simulink model "MS_QD2_QBP_joystick_R2023"  (R2023a)
settings: Solver=ode2  StartTime=0.0  StopTime=inf  FixedStep=0.001  RelTol=1e-3  EnableMultiTasking=on
undefined symbols (not defined in the file): Host, qc_get_step_size
libraries: quarc_library x67, simulink x9, simulink_extras x1
(part 2 of 2)

== system MS_QD2_QBP_joystick_R2023/MISSION SERVER LEADER FOLLOWER CONTROL/JOYSTICK_FRSKY/Pulse Check ==
  note: For this subsystem we will count the number of new pulses. The data can be considered enabled once the count of new signals has gone beyond 2. This will enable the Initializing and conditioning subsystem.
  new : Inport
  Compare : quarc_library/Logic Operations/Compare  operator=>=  output_data_type=boolean
      settings: SourceProductName=QUARC Targets
  Pulse Check : Constant
  "pulse count " : Subsystem  TreatAsAtomicUnit=on
  signal enable : Outport  InitialOutput=0  VectorParamsAs1DForOutWhenUnconnected=off
  wires:
  Compare/1 -> signal enable/1
  Pulse Check/1 -> Compare/2
  new/1 -> "pulse count "/Trigger
  "pulse count "/1(Number of Pulses) -> Compare/1

== system MS_QD2_QBP_joystick_R2023/MISSION SERVER LEADER FOLLOWER CONTROL/StopAllSignal/Subsystem ==
  Signal : Inport
  Delay : Delay  DelayLength=4
  Stop with Message : quarc_library/Sinks/Error Handling/Stop with Message  message_type=Fixed error message  message_icon=Error  message=QDrone Stopped, Stop all Models
  Threshold : quarc_library/Discontinuities/Threshold  operator=>=  param_src=Specify via dialog  threshold=0.5  duration=1
      settings: SourceProductName=QUARC Targets
  Threshold1 : quarc_library/Discontinuities/Threshold  operator=>=  param_src=Specify via dialog  threshold=0.5  duration=.3
      settings: SourceProductName=QUARC Targets
  Triggered Subsystem1 : Subsystem  TreatAsAtomicUnit=on
  Triggered Subsystem2 : Subsystem  TreatAsAtomicUnit=on
  Stop : Outport
  wires:
  Triggered Subsystem2/1(StopAllModels) -> Stop/1
  Signal/1 -> Threshold1/1, Threshold/1
  Threshold1/1 -> Triggered Subsystem2/Trigger
  Threshold/1 -> Triggered Subsystem1/Trigger, Delay/1
  Delay/1 -> Stop with Message/1

== system MS_QD2_QBP_joystick_R2023/MISSION SERVER LEADER FOLLOWER CONTROL/StopAllSignal/Subsystem1 ==
  Signal : Inport
  Delay : Delay  DelayLength=4
  Stop with Message : quarc_library/Sinks/Error Handling/Stop with Message  message_type=Fixed error message  message_icon=Error  message=Joystick triggers not back
  Threshold : quarc_library/Discontinuities/Threshold  operator=>=  param_src=Specify via dialog  threshold=0.5  duration=3
      settings: SourceProductName=QUARC Targets
  Threshold1 : quarc_library/Discontinuities/Threshold  operator=>=  param_src=Specify via dialog  threshold=0.5  duration=2
      settings: SourceProductName=QUARC Targets
  Triggered Subsystem1 : Subsystem  TreatAsAtomicUnit=on
  Triggered Subsystem2 : Subsystem  TreatAsAtomicUnit=on
  Stop : Outport
  wires:
  Triggered Subsystem2/1(StopAllModels) -> Stop/1
  Signal/1 -> Threshold1/1, Threshold/1
  Threshold1/1 -> Triggered Subsystem2/Trigger
  Threshold/1 -> Triggered Subsystem1/Trigger, Delay/1
  Delay/1 -> Stop with Message/1

== system MS_QD2_QBP_joystick_R2023/MISSION SERVER LEADER FOLLOWER CONTROL/StopAllSignal/Subsystem2 ==
  Signal : Inport
  Delay : Delay  DelayLength=4
  Stop with Message : quarc_library/Sinks/Error Handling/Stop with Message  message_type=Fixed error message  message_icon=Error  message=Not Tracking on start
  Threshold : quarc_library/Discontinuities/Threshold  operator=>=  param_src=Specify via dialog  threshold=0.5  duration=4
      settings: SourceProductName=QUARC Targets
  Threshold1 : quarc_library/Discontinuities/Threshold  operator=>=  param_src=Specify via dialog  threshold=0.5  duration=3
      settings: SourceProductName=QUARC Targets
  Triggered Subsystem1 : Subsystem  TreatAsAtomicUnit=on
  Triggered Subsystem2 : Subsystem  TreatAsAtomicUnit=on
  Stop : Outport
  wires:
  Triggered Subsystem2/1(StopAllModels) -> Stop/1
  Signal/1 -> Threshold1/1, Threshold/1
  Threshold1/1 -> Triggered Subsystem2/Trigger
  Threshold/1 -> Triggered Subsystem1/Trigger, Delay/1
  Delay/1 -> Stop with Message/1

== system MS_QD2_QBP_joystick_R2023/MISSION SERVER LEADER FOLLOWER CONTROL/StopAllSignal/Subsystem3 ==
  Signal : Inport
  Delay : Delay  DelayLength=4
  Stop with Message : quarc_library/Sinks/Error Handling/Stop with Message  message_type=Fixed error message  message_icon=Error  message=Emergency stop triggered
  Threshold : quarc_library/Discontinuities/Threshold  operator=>=  param_src=Specify via dialog  threshold=0.5  duration=2
      settings: SourceProductName=QUARC Targets
  Threshold1 : quarc_library/Discontinuities/Threshold  operator=>=  param_src=Specify via dialog  threshold=0.5  duration=.5
      settings: SourceProductName=QUARC Targets
  Triggered Subsystem1 : Subsystem  TreatAsAtomicUnit=on
  Triggered Subsystem2 : Subsystem  TreatAsAtomicUnit=on
  Stop : Outport
  wires:
  Triggered Subsystem2/1(StopAllModels) -> Stop/1
  Signal/1 -> Threshold1/1, Threshold/1
  Threshold1/1 -> Triggered Subsystem2/Trigger
  Threshold/1 -> Triggered Subsystem1/Trigger, Delay/1
  Delay/1 -> Stop with Message/1

== system MS_QD2_QBP_joystick_R2023/MISSION SERVER LEADER FOLLOWER CONTROL/StopAllSignal/Subsystem4 ==
  Signal : Inport
  Delay : Delay  DelayLength=4
  Stop with Message : quarc_library/Sinks/Error Handling/Stop with Message  message_type=Fixed error message  message_icon=Error  message=Autoland Triggered
  Threshold : quarc_library/Discontinuities/Threshold  operator=>=  param_src=Specify via dialog  threshold=0.5  duration=1
      settings: SourceProductName=QUARC Targets
  Threshold1 : quarc_library/Discontinuities/Threshold  operator=>=  param_src=Specify via dialog  threshold=0.5  duration=.3
      settings: SourceProductName=QUARC Targets
  Threshold2 : quarc_library/Discontinuities/Threshold  operator=>=  param_src=Specify via dialog  threshold=0.5  duration=10
      settings: SourceProductName=QUARC Targets
  Triggered Subsystem1 : Subsystem  TreatAsAtomicUnit=on
  Triggered Subsystem2 : Subsystem  TreatAsAtomicUnit=on
  Triggered Subsystem3 : Subsystem  TreatAsAtomicUnit=on
  Stop : Outport
  wires:
  Triggered Subsystem2/1(StopAllModels) -> Stop/1
  Threshold2/1 -> Threshold1/1, Threshold/1
  Threshold1/1 -> Triggered Subsystem2/Trigger
  Threshold/1 -> Triggered Subsystem1/Trigger, Delay/1
  Signal/1 -> Triggered Subsystem3/Trigger
  Triggered Subsystem3/1(Autoland Triggered) -> Threshold2/1
  Delay/1 -> Stop with Message/1

== system MS_QD2_QBP_joystick_R2023/MISSION SERVER LEADER FOLLOWER CONTROL/StopAllSignal/Subsystem5 ==
  Signal : Inport
  Delay : Delay  DelayLength=4
  Stop with Message : quarc_library/Sinks/Error Handling/Stop with Message  message_type=Fixed error message  message_icon=Error  message=Robots not looking towards the wall
  Threshold : quarc_library/Discontinuities/Threshold  operator=>=  param_src=Specify via dialog  threshold=0.5  duration=2
      settings: SourceProductName=QUARC Targets
  Threshold1 : quarc_library/Discontinuities/Threshold  operator=>=  param_src=Specify via dialog  threshold=0.5  duration=1
      settings: SourceProductName=QUARC Targets
  Triggered Subsystem1 : Subsystem  TreatAsAtomicUnit=on
  Triggered Subsystem2 : Subsystem  TreatAsAtomicUnit=on
  Stop : Outport
  wires:
  Triggered Subsystem2/1(StopAllModels) -> Stop/1
  Signal/1 -> Threshold1/1, Threshold/1
  Threshold1/1 -> Triggered Subsystem2/Trigger
  Threshold/1 -> Triggered Subsystem1/Trigger, Delay/1
  Delay/1 -> Stop with Message/1

== system MS_QD2_QBP_joystick_R2023/MISSION SERVER LEADER FOLLOWER CONTROL/Subsystem5/Triggered Subsystem1 ==
  Time (s) : Inport
  Trigger : TriggerPort  VariantControl=(inherit)
  Print2 : quarc_library/User Interface/Standard I//O/Print  format_string=[ %lf ] (s): DRONE ARMED \n  max_code_units=512  optimization=Minimizing latency  sample_time=-1  active=off
      settings: SourceProductName=QUARC Targets
  Terminator : Terminator
  Terminator1 : Terminator
  wires:
  Print2/2 -> Terminator/1
  Print2/1 -> Terminator1/1
  Time (s)/1 -> Print2/1

== system MS_QD2_QBP_joystick_R2023/MISSION SERVER LEADER FOLLOWER CONTROL/Subsystem5/Triggered Subsystem2 ==
  Time (s) : Inport
  Trigger : TriggerPort  VariantControl=(inherit)
  Print2 : quarc_library/User Interface/Standard I//O/Print  format_string=[ %lf ] (s): DRONE TAKEOFF \n  max_code_units=512  optimization=Minimizing latency  sample_time=-1  active=off
      settings: SourceProductName=QUARC Targets
  Terminator : Terminator
  Terminator1 : Terminator
  wires:
  Time (s)/1 -> Print2/1
  Print2/1 -> Terminator1/1
  Print2/2 -> Terminator/1

== system MS_QD2_QBP_joystick_R2023/MISSION SERVER LEADER FOLLOWER CONTROL/Subsystem5/Triggered Subsystem3 ==
  Time (s) : Inport
  Trigger : TriggerPort  VariantControl=(inherit)
  Print2 : quarc_library/User Interface/Standard I//O/Print  format_string=[ %lf ] (s): EMERGENCY STOP TRIGGERED \n  max_code_units=512  optimization=Minimizing latency  sample_time=-1  active=off
      settings: SourceProductName=QUARC Targets
  Terminator : Terminator
  Terminator1 : Terminator
  wires:
  Time (s)/1 -> Print2/1
  Print2/1 -> Terminator1/1
  Print2/2 -> Terminator/1

== system MS_QD2_QBP_joystick_R2023/MISSION SERVER LEADER FOLLOWER CONTROL/Subsystem5/Triggered Subsystem4 ==
  Time (s) : Inport
  Trigger : TriggerPort  VariantControl=(inherit)
  Print2 : quarc_library/User Interface/Standard I//O/Print  format_string=[ %lf ] (s): JOYSTICK ISSUE \n  max_code_units=512  optimization=Minimizing latency  sample_time=-1  active=off
      settings: SourceProductName=QUARC Targets
  Terminator : Terminator
  Terminator1 : Terminator
  wires:
  Print2/1 -> Terminator1/1
  Print2/2 -> Terminator/1
  Time (s)/1 -> Print2/1

== system MS_QD2_QBP_joystick_R2023/MISSION SERVER LEADER FOLLOWER CONTROL/Subsystem5/Triggered Subsystem5 ==
  Time (s) : Inport
  Trigger : TriggerPort  VariantControl=(inherit)
  Print2 : quarc_library/User Interface/Standard I//O/Print  format_string=[ %lf ] (s): START FOLLOWING \n  max_code_units=512  optimization=Minimizing latency  sample_time=-1  active=off
      settings: SourceProductName=QUARC Targets
  Terminator : Terminator
  Terminator1 : Terminator
  wires:
  Time (s)/1 -> Print2/1
  Print2/2 -> Terminator/1
  Print2/1 -> Terminator1/1

== system MS_QD2_QBP_joystick_R2023/MISSION SERVER LEADER FOLLOWER CONTROL/Subsystem5/Triggered Subsystem6 ==
  Time (s) : Inport
  Trigger : TriggerPort  TriggerType=falling  VariantControl=(inherit)
  Print2 : quarc_library/User Interface/Standard I//O/Print  format_string=[ %lf ] (s): STOP FOLLOWING \n  max_code_units=512  optimization=Minimizing latency  sample_time=-1  active=off
      settings: SourceProductName=QUARC Targets
  Terminator : Terminator
  Terminator1 : Terminator
  wires:
  Time (s)/1 -> Print2/1
  Print2/2 -> Terminator/1
  Print2/1 -> Terminator1/1

== system MS_QD2_QBP_joystick_R2023/MISSION SERVER LEADER FOLLOWER CONTROL/Subsystem5/Triggered Subsystem7 ==
  Time (s) : Inport
  Trigger : TriggerPort  TriggerType=falling  VariantControl=(inherit)
  Print2 : quarc_library/User Interface/Standard I//O/Print  format_string=[ %lf ] (s): DRONE LANDING \n  max_code_units=512  optimization=Minimizing latency  sample_time=-1  active=off
      settings: SourceProductName=QUARC Targets
  Terminator : Terminator
  Terminator1 : Terminator
  wires:
  Time (s)/1 -> Print2/1
  Print2/1 -> Terminator1/1
  Print2/2 -> Terminator/1

== system MS_QD2_QBP_joystick_R2023/MISSION SERVER LEADER FOLLOWER CONTROL/JOYSTICK_FRSKY/Pulse Check/pulse count  ==
  Trigger : TriggerPort  VariantControl=Variant
  Constant1 : Constant  Value=0
  Increment Stored Integer : simulink/Additional Math & Discrete/Additional Math: Increment - Decrement/Increment Stored Integer
  Sum : Sum  Inputs=|++
  Unit Delay : UnitDelay  SampleTime=-1  HasFrameUpgradeWarning=on
  Number of Pulses : Outport  VectorParamsAs1DForOutWhenUnconnected=off
  wires:
  Constant1/1 -> Sum/1
  Sum/1 -> Increment Stored Integer/1
  Unit Delay/1 -> Sum/2
  Increment Stored Integer/1 -> Unit Delay/1, Number of Pulses/1

== system MS_QD2_QBP_joystick_R2023/MISSION SERVER LEADER FOLLOWER CONTROL/StopAllSignal/Subsystem/Triggered Subsystem1 ==
  Trigger : TriggerPort  VariantControl=(inherit)
  Print : quarc_library/User Interface/Standard I//O/Print  format_string="Communication with QDrone Stopped, stopping all models  \\n"  max_code_units=512  optimization=Minimizing latency  sample_time=-1  active=off
      settings: SourceProductName=QUARC Targets

== system MS_QD2_QBP_joystick_R2023/MISSION SERVER LEADER FOLLOWER CONTROL/StopAllSignal/Subsystem/Triggered Subsystem2 ==
  Trigger : TriggerPort  VariantControl=(inherit)
  Constant : Constant
  StopAllModels : Outport  InitialOutput=[0]
  wires:
  Constant/1 -> StopAllModels/1

== system MS_QD2_QBP_joystick_R2023/MISSION SERVER LEADER FOLLOWER CONTROL/StopAllSignal/Subsystem1/Triggered Subsystem1 ==
  Trigger : TriggerPort  VariantControl=(inherit)
  Print : quarc_library/User Interface/Standard I//O/Print  format_string="Joystick triggers not back - Place them away from you and run again  \\n"  max_code_units=512  optimization=Minimizing latency  sample_time=-1  active=off
      settings: SourceProductName=QUARC Targets

== system MS_QD2_QBP_joystick_R2023/MISSION SERVER LEADER FOLLOWER CONTROL/StopAllSignal/Subsystem1/Triggered Subsystem2 ==
  Trigger : TriggerPort  VariantControl=(inherit)
  Constant : Constant
  StopAllModels : Outport  InitialOutput=[0]
  wires:
  Constant/1 -> StopAllModels/1

== system MS_QD2_QBP_joystick_R2023/MISSION SERVER LEADER FOLLOWER CONTROL/StopAllSignal/Subsystem2/Triggered Subsystem1 ==
  Trigger : TriggerPort  VariantControl=(inherit)
  Print : quarc_library/User Interface/Standard I//O/Print  format_string="Not tracking on start - Make sure correct vehicles are used  \\n"  max_code_units=512  optimization=Minimizing latency  sample_time=-1  active=off
      settings: SourceProductName=QUARC Targets

== system MS_QD2_QBP_joystick_R2023/MISSION SERVER LEADER FOLLOWER CONTROL/StopAllSignal/Subsystem2/Triggered Subsystem2 ==
  Trigger : TriggerPort  VariantControl=(inherit)
  Constant : Constant
  StopAllModels : Outport  InitialOutput=[0]
  wires:
  Constant/1 -> StopAllModels/1

== system MS_QD2_QBP_joystick_R2023/MISSION SERVER LEADER FOLLOWER CONTROL/StopAllSignal/Subsystem3/Triggered Subsystem1 ==
  Trigger : TriggerPort  VariantControl=(inherit)
  Print : quarc_library/User Interface/Standard I//O/Print  format_string="Emergency stop pressed  \\n"  max_code_units=512  optimization=Minimizing latency  sample_time=-1  active=off
      settings: SourceProductName=QUARC Targets

== system MS_QD2_QBP_joystick_R2023/MISSION SERVER LEADER FOLLOWER CONTROL/StopAllSignal/Subsystem3/Triggered Subsystem2 ==
  Trigger : TriggerPort  VariantControl=(inherit)
  Constant : Constant
  StopAllModels : Outport  InitialOutput=[0]
  wires:
  Constant/1 -> StopAllModels/1

== system MS_QD2_QBP_joystick_R2023/MISSION SERVER LEADER FOLLOWER CONTROL/StopAllSignal/Subsystem4/Triggered Subsystem1 ==
  Trigger : TriggerPort  VariantControl=(inherit)
  Print : quarc_library/User Interface/Standard I//O/Print  format_string="Stopped due to drone landing  \\n"  max_code_units=512  optimization=Minimizing latency  sample_time=-1  active=off
      settings: SourceProductName=QUARC Targets

== system MS_QD2_QBP_joystick_R2023/MISSION SERVER LEADER FOLLOWER CONTROL/StopAllSignal/Subsystem4/Triggered Subsystem2 ==
  Trigger : TriggerPort  VariantControl=(inherit)
  Constant : Constant
  StopAllModels : Outport  InitialOutput=[0]
  wires:
  Constant/1 -> StopAllModels/1

== system MS_QD2_QBP_joystick_R2023/MISSION SERVER LEADER FOLLOWER CONTROL/StopAllSignal/Subsystem4/Triggered Subsystem3 ==
  Trigger : TriggerPort  TriggerType=falling  VariantControl=(inherit)
  Constant : Constant
  Autoland Triggered : Outport  InitialOutput=[0]
  wires:
  Constant/1 -> Autoland Triggered/1

== system MS_QD2_QBP_joystick_R2023/MISSION SERVER LEADER FOLLOWER CONTROL/StopAllSignal/Subsystem5/Triggered Subsystem1 ==
  Trigger : TriggerPort  VariantControl=(inherit)
  Print : quarc_library/User Interface/Standard I//O/Print  format_string=One of the vehicles not placed correctly. Camera should look at back wall. \n  max_code_units=512  optimization=Minimizing latency  sample_time=-1  active=off
      settings: SourceProductName=QUARC Targets

== system MS_QD2_QBP_joystick_R2023/MISSION SERVER LEADER FOLLOWER CONTROL/StopAllSignal/Subsystem5/Triggered Subsystem2 ==
  Trigger : TriggerPort  VariantControl=(inherit)
  Constant : Constant
  StopAllModels : Outport  InitialOutput=[0]
  wires:
  Constant/1 -> StopAllModels/1

== matlab function MS_QD2_QBP_joystick_R2023/MISSION SERVER LEADER FOLLOWER CONTROL/QBotData/Extract Object Data ==
  data: data input; position output; orientation output; index input; tracking output
function [position, orientation, tracking] = fcn(data, index)

n = length(data)/7;

if (index<=0)||(index>n)
    position = zeros(1,3); orientation = zeros(1,3); tracking = 0;
else
    position = [data(index*7 -6) data(index*7 -5) data(index*7 -4)];
    orientation = [data(index*7 -3) data(index*7 -2) data(index*7 -1)];
    tracking = data(index*7);
end

== matlab function MS_QD2_QBP_joystick_R2023/MISSION SERVER LEADER FOLLOWER CONTROL/QDroneData/Extract Object Data ==
  data: data input; position output; orientation output; index input; tracking output

function [position, orientation, tracking] = fcn(data, index)

n = length(data)/7;


% position = data((index-1)*3 + 1: (index-1)*3 + 3);
% orientation = data( 3*n + 3*(index-1) + 1: 3*n + 3*(index-1) + 3);
% tracking = data(end-n+index - 1);


if (index<=0)||(index>n)
    position = zeros(1,3); orientation = zeros(1,3); tracking = 0;
else
    position = [data(index*7 -6) data(index*7 -5) data(index*7 -4)];
    orientation = [data(index*7 -3) data(index*7 -2) data(index*7 -1)];
    tracking = data(index*7);
end

== matlab function MS_QD2_QBP_joystick_R2023/Communication/Detect Communication loss/MATLAB Function ==
  data: time input; stream_connection_loss output; state input; error input
function stream_connection_loss  = fcn(time, state, error)

stream_connection_loss = 0;
if time > 1
    if ~((state == 2)&&(error >= 0))
        % stream connection is not established correctly
        stream_connection_loss = 1;
    end
end
